simulink model "x_constante"  (R2017b)
settings: Solver=VariableStepAuto  StartTime=0.0  StopTime=30000  RelTol=1e-3
values from neighbouring files (symbols this model uses):
  k1 = sym2poly(Ff_lo * Flo_xl)/a    [Xcte.m]
  k2 = sym2poly(Ff_li)/a    [Xcte.m]
  k3 = sym2poly(Ff_lo * Flo_p)/a    [Xcte.m]
  k4 = sym2poly(Fg_li) /den    [Xcte.m]
  k5 = sym2poly(Fg_gi)/den    [Xcte.m]
  k6 = sym2poly(Fg_lo* Flo_xl) /den    [Xcte.m]
  k7 = sym2poly((Fg_lo* Flo_hl)+(Fg_vl*Fvl_hl))/den    [Xcte.m]
  k8 = sym2poly(Fg_go* Fgo_xg) /den    [Xcte.m]
  k9 = sym2poly(Fg_go* Fgo_t) /den    [Xcte.m]
  tau1 = 1/a    [Xcte.m]
  tau2 = 1/a    [Xcte.m]
  tau3 = tau1    [Xcte.m]
  tau4 = 1 /den    [Xcte.m]
  tau5 = tau4    [Xcte.m]
  tau6 = tau4    [Xcte.m]
  tau7 = tau4    [Xcte.m]
  tau8 = tau4    [Xcte.m]
  tau9 = tau4    [Xcte.m]
settings Model: Creator=Rafael Azambuja  LastModifiedBy=Rafael Azambuja

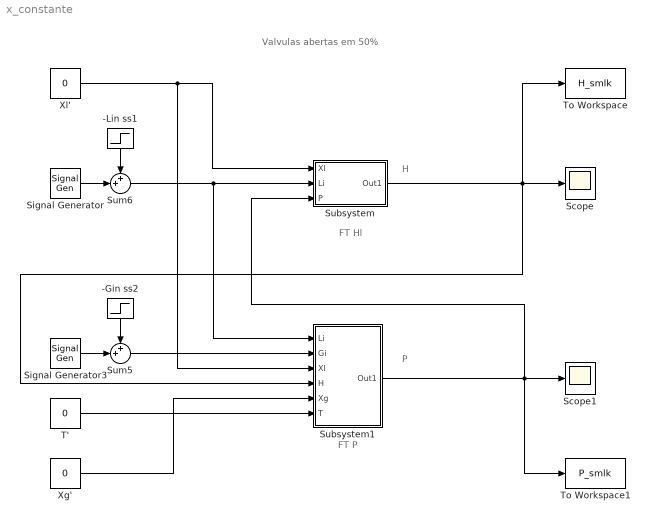
== system x_constante ==
  note: Valvulas abertas em 50%
  note: FT P
  note: FT Hl
  note: P
  note: H
  -Gin ss2 : Step  Time=0  After=0  SampleTime=0
  -Lin ss1 : Step  Time=0  After=0  SampleTime=0
  Scope : Scope
  Scope1 : Scope
  Signal Generator : SignalGenerator  Amplitude=0.05  Frequency=1/1320
  Signal Generator3 : SignalGenerator  Amplitude=0.0928  Frequency=1/1320
  Subsystem : Subsystem
  Subsystem1 : Subsystem
  Sum5 : Sum  Inputs=++|
  Sum6 : Sum  Inputs=++|
  T' : Constant  Value=0
  To Workspace : ToWorkspace  VariableName=H_smlk  SaveFormat=Timeseries  SampleTime=1
  To Workspace1 : ToWorkspace  VariableName=P_smlk  SaveFormat=Timeseries  SampleTime=1
  Xg' : Constant  Value=0
  Xl' : Constant  Value=0
  wires:
  Xg'/1 -> Subsystem1/5(Xg)
  T'/1 -> Subsystem1/6(T)
  Subsystem/1(Out1) -> To Workspace/1, Scope/1, Subsystem1/4(H)
  Subsystem1/1(Out1) -> To Workspace1/1, Scope1/1, Subsystem/3(P)
  Xl'/1 -> Subsystem1/3(Xl), Subsystem/1(Xl)
  -Lin ss1/1 -> Sum6/1
  Signal Generator/1 -> Sum6/2
  Sum6/1 -> Subsystem1/1(Li), Subsystem/2(Li)
  -Gin ss2/1 -> Sum5/1
  Signal Generator3/1 -> Sum5/2
  Sum5/1 -> Subsystem1/2(Gi)

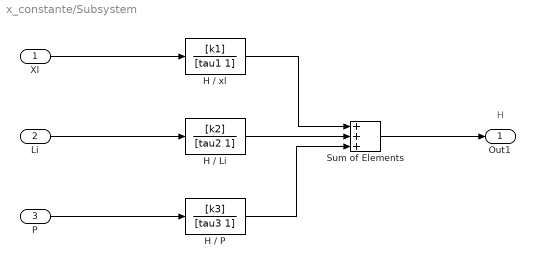
== system x_constante/Subsystem ==
  note: H
  Xl : Inport
  Li : Inport  Port=2
  P : Inport  Port=3
  H / Li : TransferFcn  Numerator=[k2]  Denominator=[tau2 1]
  H / P : TransferFcn  Numerator=[k3]  Denominator=[tau3 1]
  H / xl : TransferFcn  Numerator=[k1]  Denominator=[tau1 1]
  Sum of Elements : Sum  Inputs=+++
  Out1 : Outport
  wires:
  Xl/1 -> H / xl/1
  Li/1 -> H / Li/1
  P/1 -> H / P/1
  H / xl/1 -> Sum of Elements/1
  H / Li/1 -> Sum of Elements/2
  H / P/1 -> Sum of Elements/3
  Sum of Elements/1 -> Out1/1

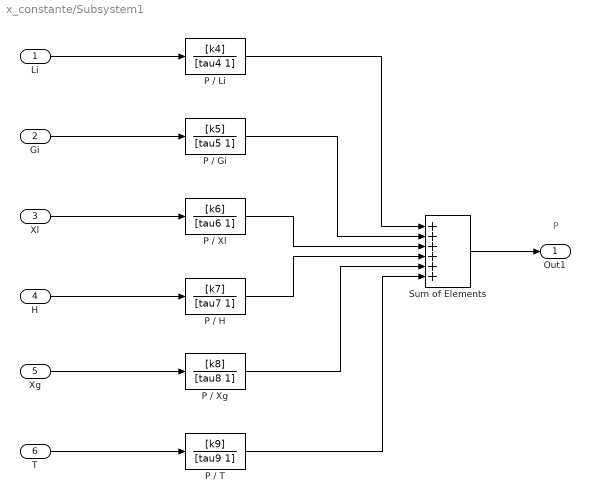
== system x_constante/Subsystem1 ==
  note: P
  Li : Inport
  Gi : Inport  Port=2
  Xl : Inport  Port=3
  H : Inport  Port=4
  Xg : Inport  Port=5
  T : Inport  Port=6
  P / Gi : TransferFcn  Numerator=[k5]  Denominator=[tau5 1]
  P / H : TransferFcn  Numerator=[k7]  Denominator=[tau7 1]
  P / Li : TransferFcn  Numerator=[k4]  Denominator=[tau4 1]
  P / T : TransferFcn  Numerator=[k9]  Denominator=[tau9 1]
  P / Xg : TransferFcn  Numerator=[k8]  Denominator=[tau8 1]
  P / Xl : TransferFcn  Numerator=[k6]  Denominator=[tau6 1]
  Sum of Elements : Sum  Inputs=++++++
  Out1 : Outport
  wires:
  Li/1 -> P / Li/1
  Gi/1 -> P / Gi/1
  Xl/1 -> P / Xl/1
  Sum of Elements/1 -> Out1/1
  H/1 -> P / H/1
  Xg/1 -> P / Xg/1
  T/1 -> P / T/1
  P / T/1 -> Sum of Elements/6
  P / Xg/1 -> Sum of Elements/5
  P / H/1 -> Sum of Elements/4
  P / Xl/1 -> Sum of Elements/3
  P / Gi/1 -> Sum of Elements/2
  P / Li/1 -> Sum of Elements/1
